simulink model "SIM_EXP3"  (R2022a)
settings: Solver=VariableStepAuto  StartTime=0.0  StopTime=1  RelTol=1e-3
values from neighbouring files (symbols this model uses):
  fct = threshold(i)    [EXP3.m]
settings Model: Creator=Dell  LastModifiedBy=Dell

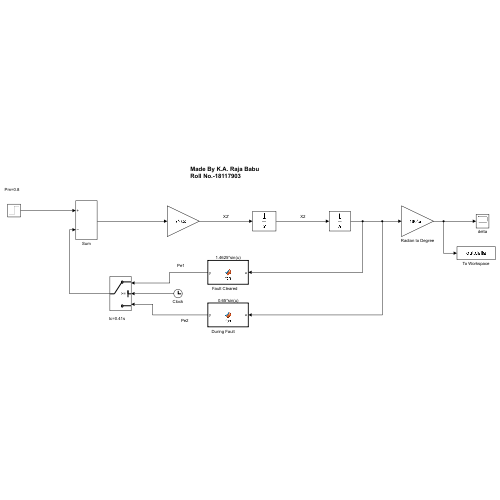
[thumbnail: Simulink's stored preview of the top-level diagram]
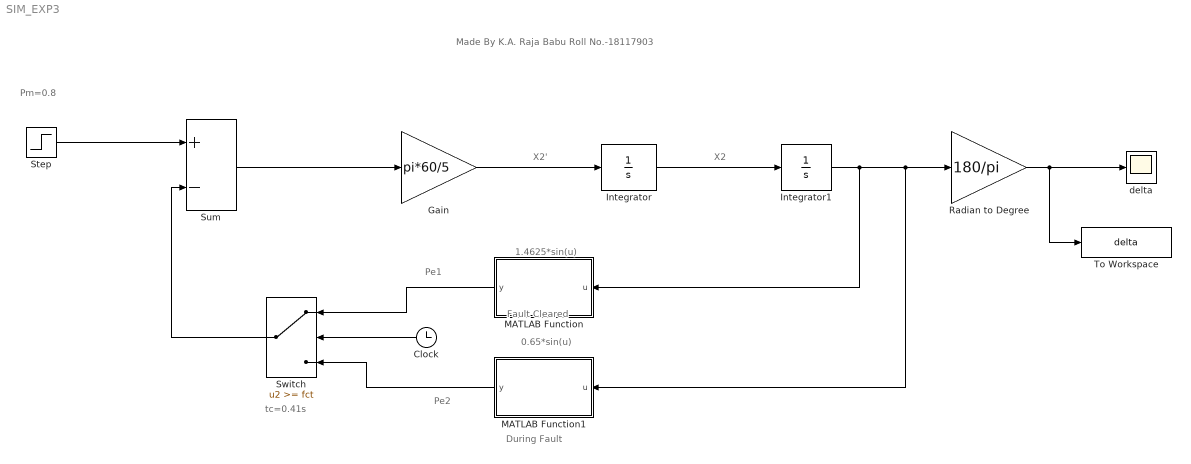
== system SIM_EXP3 ==
  note: 0.65*sin(u)
  note: 1.4625*sin(u)
  note: X2
  note: X2'
  note: tc=0.41s
  note: Pe2
  note: Pe1
  note: Made By K.A. Raja Babu
      | Roll No.-18117903
  note: During Fault
  note: Fault Cleared
  note: Pm=0.8
  Clock : Clock
      settings: Decimation=1000
  Gain : Gain  Gain=pi*60/5
  Integrator : Integrator
  Integrator1 : Integrator  InitialCondition=0.46055
  MATLAB Function : MATLAB Function  TreatAsAtomicUnit=on
  MATLAB Function1 : MATLAB Function  TreatAsAtomicUnit=on
  Radian to Degree : Gain  Gain=180/pi
  Step : Step  Time=10  Before=0.8  SampleTime=0
  Sum : Sum  Inputs=+-
  Switch : Switch  Threshold=fct  SaturateOnIntegerOverflow=off  InputSameDT=off
  To Workspace : ToWorkspace  VariableName=delta  SampleTime=-1
  delta : Scope
  wires:
  Sum/1 -> Gain/1
  Gain/1 -> Integrator/1
  Integrator/1 -> Integrator1/1
  Step/1 -> Sum/1
  Clock/1 -> Switch/2
  MATLAB Function1/1(y) -> Switch/3
  MATLAB Function/1(y) -> Switch/1
  Switch/1 -> Sum/2
  Integrator1/1 -> MATLAB Function/1(u), Radian to Degree/1, MATLAB Function1/1(u)
  Radian to Degree/1 -> To Workspace/1, delta/1

== matlab function SIM_EXP3/MATLAB Function ==
  data: u input; y output
function y = fcn(u)

y = 1.4625*sin(u);

== matlab function SIM_EXP3/MATLAB Function1 ==
  data: u input; y output
function y = fcn(u)

y = 0.65*sin(u);
